simulink model "stacked_singleEMRAX_angleChange"  (R2021a)
settings: Solver=ode45  StartTime=0.0  StopTime=20  RelTol=1e-4  EnableMultiTasking=on
InitFcn:
  | %Atmospheric Properties
  | rho_air = 1.2754;  % air density in kg/m^3
  | mu = 1.803e-5; % dynamic viscosity [N-s/m^2]
  | 
  | Vbus = 175;  % Actual bus voltage (volts) that will be applied
  | % Emrax 208
  | R = .0122;  %  resistance, ohms, line-line at room temp
  | L = 125*10^-6;  %  inductance line-line at commutation frequency, henries
  | t_elec = L/R;
  | 
  | Irotor = 256/100^2;  %  kg*m^2 -- From Emrax data sheet
  | Kt_motor = .80;  %  N*m/Arms
  | Ke_motor = .0487*sqrt(2)*60/(2*pi);  %  Vpk/rad/sec
  | Ke = .0487*sqrt(2)*60/(2*pi);   %radians/sec
  | 
  | CurrentSenseMax = 250;  %  Max current sense from controller code
  | BASE_CURRENT = 125;   %  Max current in amps corresponding to normalized control loop current = 1
  | LOOP_FREQUENCY = 35;     % in kHz
  | T_LOOP = .001/LOOP_FREQUENCY;
  | pwm_loop_prescalar = 1;  %Presacalar how many PWM cycles for one current loop execution
  | T_PWM = T_LOOP/pwm_loop_prescalar;  %  Current loop prescaler on PWM is 1 for Uber
  | POLES = 20;
  | BASE_FREQ = 1200; %POLES/2*1300/60;  %  1300 rpm
  | BaseSpeed     = BASE_FREQ*(60.0/(POLES/2.0));
  | 
  | % current loop
  | alpha = 250*2*pi;         % current loop bandwidth
  | 
  | omega = 0;               % omega for de-coupling integrator
  | 
  | % Current loop
  | %          Motor_Params.ILOOP_BW = (2*PI*1000.0);
  | %        Motor_Params.id_KP = Motor_Params.ILOOP_BW*Motor_Params.StatorInductance;
  | %      Motor_Params.id_KI = Motor_Params.ILOOP_BW*Motor_Params.StatorResistance;
  | %      Motor_Params.iq_KP = Motor_Params.ILOOP_BW*Motor_Params.StatorInductance;
  | %     Motor_Params.iq_KI = Motor_Params.ILOOP_BW*Motor_Params.StatorResistance;
  | I_Kp = alpha*L*1;
  | I_Ki = alpha*R/I_Kp*T_LOOP;
  | %I_Ki = alpha*R*0;
  | 
  | % Speed loop
  | SpeedLoopPrescale = 5;
  | Tspeedloop = T_LOOP*SpeedLoopPrescale;
  | PID_spd_Kp = 3;   % From Uber code (ORIGINIAL: 3)
  | PID_spd_Ki = .15*Tspeedloop*1.5;   % From Uber code (ORIGINAL: 0.15*Tspeedloop*2)
  | 
  | Ramp_secs = 100;    %  Ramp slew rate limiter, this number is the number of seconds to ramp from 0 to basespeed
  | 
  | % Position loop
  | speedErrorPEngage = .003; % Speed error max for position loop to enable
  | % Code has .001 for PEngage, trying something diff here
  | PID_pos_Kp = .25;
  | PID_pos_Ki = .00003;
  | PID_pos_Kd = 20000;
  | 
  | PID_pos_error_sat = .3;  % Maximum error saturated into position PID (in simulink, not C right now)
  | PID_pos_sat = .25;  %  From code, based on DC bus limit
  | PID_pos_C1 = 1; %  Position loop D bandlimit filter
  | PID_pos_C2 = 0;  %  Position loop D bandlimit filter
  | 
  | 
  | % transfer function of speed estimator is K1*K3*z/(z-K2)
  | %  Pole is at z = K2
  | % z = exp(-sT)
  | f_estpole = 35000;
  | K1 = 1/(BASE_FREQ*T_LOOP);   %  Divide by base freq to convert from elec delta-normalized-angle/cycle to [0,1] normalized speed
  |      %  K1 converts delta angle estimate over a loop period to a [0,1] speed estimate
  | K2 = exp(-f_estpole*2*pi*T_LOOP);
  | K3 = 1 - K2;  % Set to make filter have unity gain at 0 frequency (z = 1)
  | 
  | %Blade properties
  | d_prop = 2.216;   %  diameter propeller [m]
  | Cp = 11000/rho_air/d_prop^5/(1300/60*2*pi)^3;   % 11000 W at 1300 rpm static thrust
  | cla = 5.73; %local lift slope [/rad] ASSUMED CONSTANT
  | cd = 0.01; %local drag coeff. ASSUMED CONSTANT
  | c = 0.08; %chord [m]
  | nb = 2; %number of blades
  | sigma = nb*c/pi/(d_prop/2);
  | Ihub = 0.0143;
  | Iblade = 0.1275;
  | Idrive = 0.0052;
  | Iloadcell = 0.011;
  | Irotorshaft = 0.0076;
  | GR = 1.6; %gear ratio
  | Ielements = Ihub*2 + Iblade*nb + Iloadcell*2;
  | I_eff = Ielements*(1/GR)^2;
  | Iload = I_eff + Idrive;   % .33 Jayant email 3/6/2019 ;  .2 jayant email 7/11/2018
  | 
  | 
  | 
  | InitialRPM = 1920;
  | omegamech = InitialRPM/60*2*pi;  %  Used to preload Q current voltage integrator
  | 
  | % Serial Message frequency (messages per second)
  | MsgFreq = 1000;
undefined symbols (not defined in the file): DiscIntNeverNeededParam, magnitude
settings Model: ModifiedHistory=4/7/2020 Adding in voltage saturation to mag 1 before SVGEN  Creator=mricci  LastModifiedBy=asper101
settings SolverCC: AlgebraicLoopSolver=TrustRegion
settings DataIOCC: LimitDataPoints=on  SaveFormat=Array  SignalLoggingSaveFormat=ModelDataLogs  ReturnWorkspaceOutputs=off
settings OptimizationCC: ExpressionDepthLimit=2147483647  InitFltsAndDblsToZero=on  LifeSpan=inf
settings DebuggingCC: UnderspecifiedInitializationDetection=Classic  MergeDetectMultiDrivingBlocksExec=none  SolverPrmCheckMsg=warning  FcnCallInpInsideContextMsg=warning  StateNameClashWarn=warning  SFUnexpectedBacktrackingDiag=warning  SFNoUnconditionalDefaultTransitionDiag=warning  SFExecutionAtInitializationDiag=none  SFMachineParentedDataDiag=warning  ArithmeticOperatorsInVariantConditions=warning
settings HardwareCC: ProdBitPerPointer=32  ProdBitPerSizeT=32  ProdBitPerPtrDiffT=32  ProdLargestAtomicFloat=None  ProdIntDivRoundTo=Undefined  ProdEndianess=Unspecified  ProdWordSize=32  ProdHWDeviceType=32-bit Generic
settings ModelReferenceCC: PropagateSignalLabelsOutOfModel=off
settings CodeAppCC: StateflowObjectComments=on
settings GRTTargetCC: TargetLangStandard=C89/C90 (ANSI)  CombineOutputUpdateFcns=off  GRTInterface=on
settings ConfigComp: CovMetricSettings=dw  CovSaveCumulativeToWorkspaceVar=on  CovSaveSingleToWorkspaceVar=on

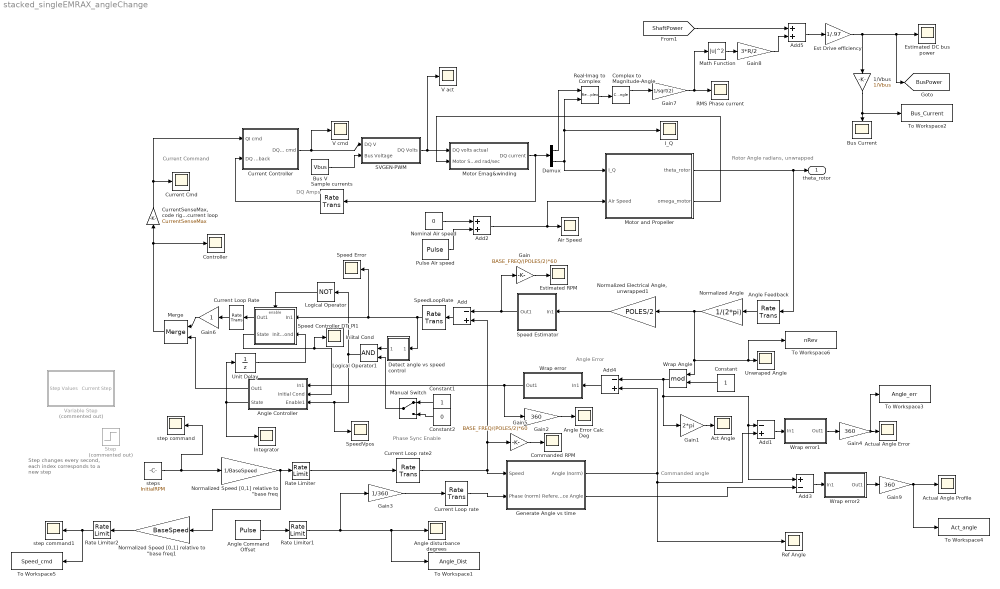
== system stacked_singleEMRAX_angleChange ==
  note: Phase Sync Enable
  note: Current Command
  note: Rotor Angle radians, unwrapped
  note: Commanded angle
  note: Angle Error
  note: DQ Amps
  note: Step changes every second, each index corresponds to a new step
  1/Vbus : Gain  Gain=1/Vbus
  Act Angle : Scope
  Actual Angle Error : Scope
  Actual Angle Profile : Scope
  Add : Sum  Inputs=-+
  Add1 : Sum  Inputs=-+
  Add2 : Sum
  Add3 : Sum  Inputs=+-
  Add4 : Sum  Inputs=-+
  Add5 : Sum
  Air Speed : Scope
  Angle Command Offset : DiscretePulseGenerator  PulseType=Time based  Amplitude=5  Period=6  PulseWidth=50  PhaseDelay=10
  Angle Controller : Subsystem  TreatAsAtomicUnit=on
  Angle Error Calc Deg : Scope
  Angle Feedback : RateTransition  OutPortSampleTime=T_LOOP
  Angle disturbance degrees : Scope
  Bus Current : Scope
  Bus V : Constant  Value=Vbus
  Commanded RPM : Scope
  Complex to Magnitude-Angle : ComplexToMagnitudeAngle
  Constant : Constant
  Constant1 : Constant
  Constant2 : Constant  Value=0
  Controller : Scope
  Current Loop Rate : RateTransition  OutPortSampleTime=T_LOOP
  Current Cmd : Scope
  Current Controller : Subsystem
  Current Loop rate : RateTransition  OutPortSampleTime=T_LOOP
  Current Loop rate2 : RateTransition  OutPortSampleTime=T_LOOP
  "CurrentSenseMax, code right now has Controller outputting PU amps then scaled to amps going into current loop" : Gain  Gain=CurrentSenseMax
  Demux : Demux  Outputs=2
  Detect angle vs speed control : Subsystem
  Est Drive efficiency : Gain  Gain=1/.97
  Estimated DC bus power : Scope
  Estimated RPM : Scope
  Gain : Gain  Gain=BASE_FREQ/(POLES/2)*60
  Gain1 : Gain  Gain=2*pi
  Gain2 : Gain  Gain=360
  Gain3 : Gain  Gain=1/360
  Gain4 : Gain  Gain=360
  Gain5 : Gain  Gain=BASE_FREQ/(POLES/2)*60
  Gain6 : Gain
  Gain7 : Gain  Gain=1/sqrt(2)
  Gain8 : Gain  Gain=3*R/2
  Gain9 : Gain  Gain=360
  Generate Angle vs time : Subsystem
  I_Q : Scope
  Iniital Cond : Scope
  Integrator : Scope
  Logical Operator : Logic  Operator=NOT  AllPortsSameDT=off  OutDataTypeStr=boolean
  Logical Operator1 : Logic  AllPortsSameDT=off  OutDataTypeStr=boolean
  Manual Switch : ManualSwitch
  Math Function : Math  Operator=magnitude^2  SaturateOnIntegerOverflow=on
  Merge : Merge
  Motor Emag&winding : Subsystem
  Motor and Propeller : Subsystem
  Nominal Air speed : Constant  Value=0
  Normalized Angle : Gain  Gain=1/(2*pi)
  "Normalized Electrical Angle, unwrapped1" : Gain  Gain=POLES/2
  "Normalized Speed [0,1] relative to \"base freq" : Gain  Gain=1/BaseSpeed
  "Normalized Speed [0,1] relative to \"base freq1" : Gain  Gain=BaseSpeed
  Pulse Air speed : DiscretePulseGenerator  PulseType=Time based  Amplitude=0  Period=6  PulseWidth=50
  RMS Phase current : Scope
  Rate Limiter : RateLimiter  RisingSlewLimit=5/Ramp_secs  FallingSlewLimit=-5/Ramp_secs  SampleTimeMode=inherited  InitialCondition=InitialRPM/BaseSpeed
  Rate Limiter1 : RateLimiter  RisingSlewLimit=5/.1  FallingSlewLimit=-5/.1  SampleTimeMode=inherited
  Rate Limiter2 : RateLimiter  RisingSlewLimit=5/Ramp_secs  FallingSlewLimit=-5/Ramp_secs  SampleTimeMode=inherited  InitialCondition=InitialRPM/BaseSpeed
  Real-Imag to Complex : RealImagToComplex
  Ref Angle : Scope
  SVGEN-PWM : Subsystem
  Sample currents : RateTransition  OutPortSampleTime=T_LOOP
  Speed Controller DT_PI1 : Subsystem
  Speed Error : Scope
  Speed Estimator : Subsystem
  SpeedLoopRate : RateTransition  OutPortSampleTime=T_LOOP*SpeedLoopPrescale
  SpeedVpos : Scope
  Step : Step  Commented=on  Time=.25  Before=InitialRPM  After=1280
  To Workspace1 : ToWorkspace  VariableName=Angle_Dist  SaveFormat=Timeseries  SampleTime=-1
  To Workspace2 : ToWorkspace  VariableName=Bus_Current  SaveFormat=Timeseries  SampleTime=-1
  To Workspace3 : ToWorkspace  VariableName=Angle_err  SaveFormat=Timeseries  SampleTime=-1
  To Workspace4 : ToWorkspace  VariableName=Act_angle  SaveFormat=Timeseries  SampleTime=-1
  To Workspace5 : ToWorkspace  VariableName=Speed_cmd  SaveFormat=Timeseries  SampleTime=-1
  To Workspace6 : ToWorkspace  VariableName=nRev  SaveFormat=Timeseries  SampleTime=-1
  Unit Delay : UnitDelay
  Unwraped Angle : Scope
  V act : Scope
  V cmd : Scope
  Variable Step : Subsystem  Commented=on
  Wrap Angle : Math  Operator=mod  SignedPower=on  SaturateOnIntegerOverflow=on
  Wrap error : Subsystem
  Wrap error1 : Subsystem
  Wrap error2 : Subsystem
  step command : Scope
  step command1 : Scope
  steps : Constant  Value=InitialRPM
  theta_rotor : Outport
  tag scope: BusPower=global
  wires:
  Motor and Propeller/1(theta_rotor) -> theta_rotor/1, Angle Feedback/1
  Add/1 -> SpeedLoopRate/1
  Speed Estimator/1(Out1) -> Add/1, Gain/1
  Add2/1 -> Air Speed/1, Motor and Propeller/2(Air Speed)
  Nominal Air speed/1 -> Add2/1
  Pulse Air speed/1 -> Add2/2
  Gain/1 -> Estimated RPM/1
  Wrap Angle/1 -> Add4/1, Gain1/1, Add3/1, Add1/1
  Constant/1 -> Wrap Angle/2
  Generate Angle vs time/1(Angle (norm)) -> Add1/2, Ref Angle/1, Add4/2
  Wrap error/1(Out1) -> Gain2/1, Angle Controller/1(In1)
  Add4/1 -> Wrap error/1(In1)
  Angle Command Offset/1 -> Rate Limiter1/1
  Speed Controller DT_PI1/1(Out1) -> Current Loop Rate/1
  Merge/1 -> "CurrentSenseMax, code right now has Controller outputting PU amps then scaled to amps going into current loop"/1, Controller/1
  SpeedLoopRate/1 -> Speed Controller DT_PI1/1(In1), Speed Error/1, Detect angle vs speed control/1(In1)
  "CurrentSenseMax, code right now has Controller outputting PU amps then scaled to amps going into current loop"/1 -> Current Controller/1(QI cmd), Current Cmd/1
  Logical Operator1/1 -> Logical Operator/1, Angle Controller/3(Enable1), SpeedVpos/1
  Motor and Propeller/2(omega_motor) -> Motor Emag&winding/2(Motor Speed rad/sec)
  Current Loop rate/1 -> Generate Angle vs time/2(Phase (norm))
  Sample currents/1 -> Current Controller/2(DQ I feedback)
  Motor Emag&winding/1(DQ current) -> Demux/1, Sample currents/1
  Demux/2 -> Real-Imag to Complex/2, I_Q/1, Motor and Propeller/1(I_Q)
  Angle Feedback/1 -> Normalized Angle/1
  Normalized Angle/1 -> "Normalized Electrical Angle, unwrapped1"/1, To Workspace6/1, Unwraped Angle/1, Wrap Angle/1
  Angle Controller/1(Out1) -> Merge/2
  "Normalized Electrical Angle, unwrapped1"/1 -> Speed Estimator/1(In1)
  Gain1/1 -> Act Angle/1
  Gain3/1 -> Current Loop rate/1
  Gain2/1 -> Angle Error Calc Deg/1
  Add1/1 -> Wrap error1/1(In1)
  Wrap error1/1(Out1) -> Gain4/1
  Gain4/1 -> To Workspace3/1, Actual Angle Error/1
  Current Loop rate2/1 -> Generate Angle vs time/1(Speed), Add/2, Gain5/1
  Angle Controller/2(State) -> Unit Delay/1, Integrator/1
  Speed Controller DT_PI1/2(State) -> Angle Controller/2(Initial Cond), Iniital Cond/1
  Gain5/1 -> Commanded RPM/1
  Current Loop Rate/1 -> Gain6/1
  Gain6/1 -> Merge/1
  Logical Operator/1 -> Speed Controller DT_PI1/Enable
  Current Controller/1(DQ V cmd) -> SVGEN-PWM/1(DQ V), V cmd/1
  SVGEN-PWM/1(DQ Volts) -> V act/1, Motor Emag&winding/1(DQ volts actual)
  Bus V/1 -> SVGEN-PWM/2(Bus Voltage)
  Unit Delay/1 -> Speed Controller DT_PI1/2(Initial Cond)
  Rate Limiter/1 -> Current Loop rate2/1
  Detect angle vs speed control/1(Out1) -> Logical Operator1/1
  Manual Switch/1 -> Logical Operator1/2
  Constant1/1 -> Manual Switch/1
  Constant2/1 -> Manual Switch/2
  "Normalized Speed [0,1] relative to \"base freq"/1 -> "Normalized Speed [0,1] relative to \"base freq1"/1, Rate Limiter/1
  Demux/1 -> Real-Imag to Complex/1
  Real-Imag to Complex/1 -> Complex to Magnitude-Angle/1
  Complex to Magnitude-Angle/1 -> Gain7/1
  Gain7/1 -> Math Function/1, RMS Phase current/1
  [ShaftPower] -> Add5/1
  Math Function/1 -> Gain8/1
  Gain8/1 -> Add5/2
  Add5/1 -> Est Drive efficiency/1
  Est Drive efficiency/1 -> 1/Vbus/1, [BusPower], Estimated DC bus power/1
  1/Vbus/1 -> To Workspace2/1, Bus Current/1
  Gain9/1 -> To Workspace4/1, Actual Angle Profile/1
  Wrap error2/1(Out1) -> Gain9/1
  Add3/1 -> Wrap error2/1(In1)
  Generate Angle vs time/2(Reference Angle) -> Add3/2
  Rate Limiter1/1 -> Gain3/1, Angle disturbance degrees/1, To Workspace1/1
  "Normalized Speed [0,1] relative to \"base freq1"/1 -> Rate Limiter2/1
  Rate Limiter2/1 -> To Workspace5/1, step command1/1
  steps/1 -> step command/1, "Normalized Speed [0,1] relative to \"base freq"/1

== system stacked_singleEMRAX_angleChange/Angle Controller ==
  In1 : Inport
  Initial Cond : Inport  Port=2
  Enable1 : Inport  Port=3
  Angle Controller DT_PID saturate P : Subsystem
  Max error : Saturate  UpperLimit=PID_pos_error_sat  LowerLimit=-PID_pos_error_sat
  Out1 : Outport  InitialOutput=[0]
  State : Outport  Port=2  InitialOutput=[0]
  wires:
  In1/1 -> Max error/1
  Max error/1 -> Angle Controller DT_PID saturate P/1(In1)
  Initial Cond/1 -> Angle Controller DT_PID saturate P/2(Iniitial Cond)
  Enable1/1 -> Angle Controller DT_PID saturate P/Enable
  Angle Controller DT_PID saturate P/1(Out1) -> Out1/1
  Angle Controller DT_PID saturate P/2(Integrator) -> State/1

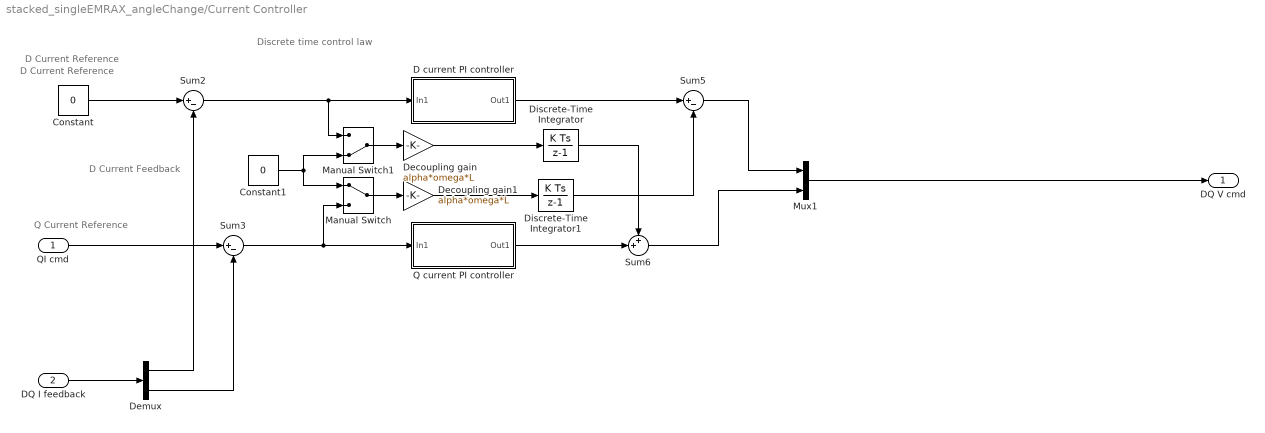
== system stacked_singleEMRAX_angleChange/Current Controller ==
  note: D Current Reference
  note: D Current Feedback
  note: D Current Reference
  note: Q Current Reference
  note: Discrete
      | time control
      | law
  QI cmd : Inport
  DQ I feedback : Inport  Port=2
  Constant : Constant  Value=0
  Constant1 : Constant  Value=0
  D current PI controller : Subsystem
  Decoupling gain : Gain  Gain=alpha*omega*L
  Decoupling gain1 : Gain  Gain=alpha*omega*L
  Demux : Demux  Outputs=2
  Discrete-Time Integrator : DiscreteIntegrator  SampleTime=T_LOOP  ICPrevOutput=DiscIntNeverNeededParam  ICPrevScaledInput=DiscIntNeverNeededParam
  Discrete-Time Integrator1 : DiscreteIntegrator  SampleTime=T_LOOP  ICPrevOutput=DiscIntNeverNeededParam  ICPrevScaledInput=DiscIntNeverNeededParam
  Manual Switch : ManualSwitch
  Manual Switch1 : ManualSwitch  CurrentSetting=0
  Mux1 : Mux  Inputs=2
  Q current PI controller : Subsystem
  Sum2 : Sum  Inputs=|+-
  Sum3 : Sum  Inputs=|+-
  Sum5 : Sum  Inputs=|+-
  Sum6 : Sum  Inputs=++|
  DQ V cmd : Outport
  wires:
  Mux1/1 -> DQ V cmd/1
  Sum2/1 -> D current PI controller/1(In1), Manual Switch1/1
  Sum3/1 -> Q current PI controller/1(In1), Manual Switch/2
  Constant/1 -> Sum2/1
  D current PI controller/1(Out1) -> Sum5/1
  Q current PI controller/1(Out1) -> Sum6/2
  Discrete-Time Integrator/1 -> Sum6/1
  Discrete-Time Integrator1/1 -> Sum5/2
  QI cmd/1 -> Sum3/1
  Decoupling gain1/1 -> Discrete-Time Integrator1/1
  Decoupling gain/1 -> Discrete-Time Integrator/1
  Manual Switch/1 -> Decoupling gain1/1
  Manual Switch1/1 -> Decoupling gain/1
  Constant1/1 -> Manual Switch1/2, Manual Switch/1
  Sum5/1 -> Mux1/1
  Sum6/1 -> Mux1/2
  DQ I feedback/1 -> Demux/1
  Demux/1 -> Sum2/2
  Demux/2 -> Sum3/2

== system stacked_singleEMRAX_angleChange/Detect angle vs speed control ==
  In1 : Inport
  Abs : Abs
  Relay : Relay  OnSwitchValue=2*speedErrorPEngage  OffSwitchValue=speedErrorPEngage  OnOutputValue=0  OffOutputValue=1
  Out1 : Outport
  wires:
  Abs/1 -> Relay/1
  In1/1 -> Abs/1
  Relay/1 -> Out1/1

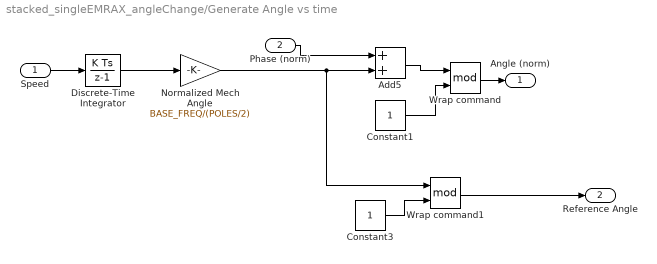
== system stacked_singleEMRAX_angleChange/Generate Angle vs time ==
  Speed : Inport
  Phase (norm) : Inport  Port=2
  Add5 : Sum
  Constant1 : Constant
  Constant3 : Constant
  Discrete-Time Integrator : DiscreteIntegrator  SampleTime=-1  ICPrevOutput=DiscIntNeverNeededParam  ICPrevScaledInput=DiscIntNeverNeededParam
  Normalized Mech Angle : Gain  Gain=BASE_FREQ/(POLES/2)
  Wrap command : Math  Operator=mod  SignedPower=on  SaturateOnIntegerOverflow=on
  Wrap command1 : Math  Operator=mod  SignedPower=on  SaturateOnIntegerOverflow=on
  Angle (norm) : Outport
  Reference Angle : Outport  Port=2
  wires:
  Constant1/1 -> Wrap command/2
  Discrete-Time Integrator/1 -> Normalized Mech Angle/1
  Add5/1 -> Wrap command/1
  Speed/1 -> Discrete-Time Integrator/1
  Phase (norm)/1 -> Add5/1
  Wrap command/1 -> Angle (norm)/1
  Constant3/1 -> Wrap command1/2
  Normalized Mech Angle/1 -> Wrap command1/1, Add5/2
  Wrap command1/1 -> Reference Angle/1

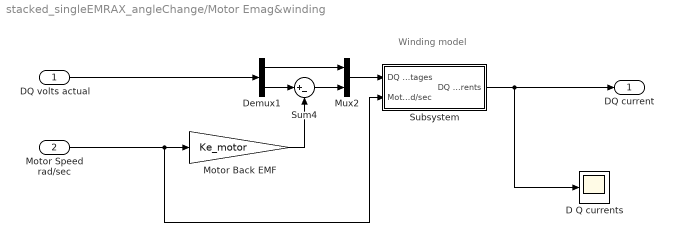
== system stacked_singleEMRAX_angleChange/Motor Emag&winding ==
  note: Winding model
  DQ volts actual : Inport
  Motor Speed rad/sec : Inport  Port=2
  D Q currents : Scope
  Demux1 : Demux  Outputs=2
  Motor Back EMF : Gain  Gain=Ke_motor
  Mux2 : Mux  Inputs=2
  Subsystem : Subsystem
  Sum4 : Sum  Inputs=|+-
  DQ current : Outport
  wires:
  Motor Speed rad/sec/1 -> Motor Back EMF/1, Subsystem/2(Motor speed rad/sec)
  Mux2/1 -> Subsystem/1(DQ voltages)
  Demux1/1 -> Mux2/1
  Demux1/2 -> Sum4/1
  Sum4/1 -> Mux2/2
  Motor Back EMF/1 -> Sum4/2
  DQ volts actual/1 -> Demux1/1
  Subsystem/1(DQ currents) -> DQ current/1, D Q currents/1

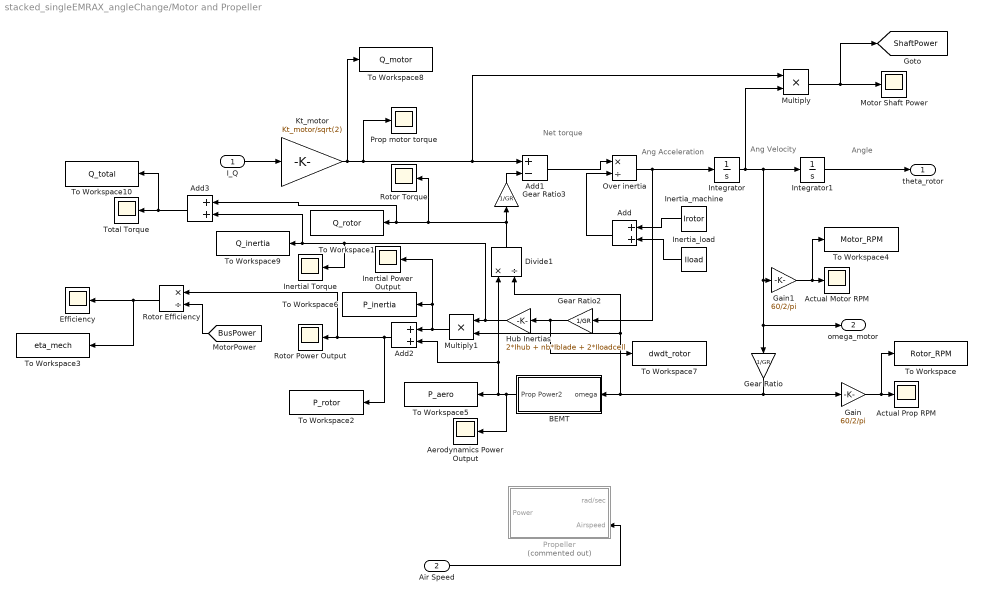
== system stacked_singleEMRAX_angleChange/Motor and Propeller ==
  note: Ang Acceleration
  note: Angle
  note: Ang Velocity
  note: Net torque
  I_Q : Inport
  Air Speed : Inport  Port=2
  Actual Motor RPM : Scope
  Actual Prop RPM : Scope
  Add : Sum
  Add1 : Sum  Inputs=+-
  Add2 : Sum
  Add3 : Sum
  Aerodynamics Power Output : Scope
  BEMT : Subsystem
  Divide1 : Product  Inputs=*/
  Efficiency : Scope
  Gain : Gain  Gain=60/2/pi
  Gain1 : Gain  Gain=60/2/pi
  Gear Ratio : Gain  Gain=1/GR
  Gear Ratio2 : Gain  Gain=1/GR
  Gear Ratio3 : Gain  Gain=1/GR
  Hub Inertias : Gain  Gain=2*Ihub + nb*Iblade + 2*Iloadcell
  Inertia_load : Constant  Value=Iload
  Inertia_machine : Constant  Value=Irotor
  Inertial Power Output : Scope
  Inertial Torque : Scope
  Integrator : Integrator  InitialCondition=InitialRPM*2*pi/60
  Integrator1 : Integrator
  Kt_motor : Gain  Gain=Kt_motor/sqrt(2)
  Motor Shaft Power : Scope
  Multiply : Product  Inputs=**
  Multiply1 : Product  Inputs=**
  Over inertia : Product  Inputs=*/
  Prop motor torque : Scope
  Propeller : Subsystem  Commented=on
  Rotor Efficiency : Product  Inputs=*/
  Rotor Power Output : Scope
  Rotor Torque : Scope
  To Workspace : ToWorkspace  VariableName=Rotor_RPM  SaveFormat=Timeseries  SampleTime=-1
  To Workspace1 : ToWorkspace  VariableName=Q_rotor  SaveFormat=Timeseries  SampleTime=-1
  To Workspace10 : ToWorkspace  VariableName=Q_total  SaveFormat=Timeseries  SampleTime=-1
  To Workspace2 : ToWorkspace  VariableName=P_rotor  SaveFormat=Timeseries  SampleTime=-1
  To Workspace3 : ToWorkspace  VariableName=eta_mech  SaveFormat=Timeseries  SampleTime=-1
  To Workspace4 : ToWorkspace  VariableName=Motor_RPM  SaveFormat=Timeseries  SampleTime=-1
  To Workspace5 : ToWorkspace  VariableName=P_aero  SaveFormat=Timeseries  SampleTime=-1
  To Workspace6 : ToWorkspace  VariableName=P_inertia  SaveFormat=Timeseries  SampleTime=-1
  To Workspace7 : ToWorkspace  VariableName=dwdt_rotor  SaveFormat=Timeseries  SampleTime=-1
  To Workspace8 : ToWorkspace  VariableName=Q_motor  SaveFormat=Timeseries  SampleTime=-1
  To Workspace9 : ToWorkspace  VariableName=Q_inertia  SaveFormat=Timeseries  SampleTime=-1
  Total Torque : Scope
  theta_rotor : Outport
  omega_motor : Outport  Port=2
  tag scope: ShaftPower=global
  wires:
  Integrator/1 -> Integrator1/1, Gain1/1, omega_motor/1, Gear Ratio/1, Multiply/2
  I_Q/1 -> Kt_motor/1
  Air Speed/1 -> Propeller/2(Airspeed)
  Over inertia/1 -> Gear Ratio2/1, Integrator/1
  Integrator1/1 -> theta_rotor/1
  Add1/1 -> Over inertia/1
  Kt_motor/1 -> Multiply/1, Add1/1, Prop motor torque/1, To Workspace8/1
  Gain/1 -> To Workspace/1, Actual Prop RPM/1
  Inertia_machine/1 -> Add/1
  Inertia_load/1 -> Add/2
  Add/1 -> Over inertia/2
  Multiply/1 -> [ShaftPower], Motor Shaft Power/1
  Gear Ratio/1 -> Divide1/2, Multiply1/2, BEMT/1(omega), Gain/1
  BEMT/1(Prop Power2) -> Aerodynamics Power Output/1, Add2/2, Divide1/1, To Workspace5/1
  Rotor Efficiency/1 -> To Workspace3/1, Efficiency/1
  Gain1/1 -> To Workspace4/1, Actual Motor RPM/1
  [BusPower] -> Rotor Efficiency/2
  Add2/1 -> Rotor Efficiency/1, Rotor Power Output/1, To Workspace2/1
  Gear Ratio2/1 -> To Workspace7/1, Hub Inertias/1
  Gear Ratio3/1 -> Add1/2
  Divide1/1 -> Rotor Torque/1, Add3/1, To Workspace1/1, Gear Ratio3/1
  Hub Inertias/1 -> Inertial Torque/1, Add3/2, To Workspace9/1, Multiply1/1
  Multiply1/1 -> Inertial Power Output/1, To Workspace6/1, Add2/1
  Add3/1 -> To Workspace10/1, Total Torque/1

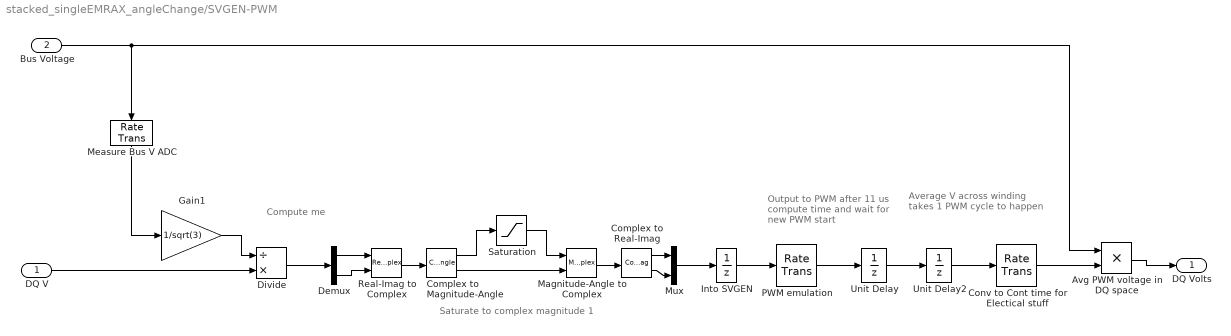
== system stacked_singleEMRAX_angleChange/SVGEN-PWM ==
  note: Saturate to complex magnitude 1
  note: Output to PWM
      | after 11 us compute time
      | and wait for new PWM start
  note: Average V
      | across winding
      | takes 1 PWM
      | cycle to happen
  note: Compute
      | me
  DQ V : Inport
  Bus Voltage : Inport  Port=2
  Avg PWM voltage in DQ space : Product  RndMeth=Zero
  Complex to Magnitude-Angle : ComplexToMagnitudeAngle
  Complex to Real-Imag : ComplexToRealImag
  Conv to Cont time for Electical stuff : RateTransition
  Demux : Demux  Outputs=2
  Divide : Product  Inputs=/*
  Gain1 : Gain  Gain=1/sqrt(3)
  Into SVGEN : UnitDelay  InitialCondition=[ 0 ; omegamech*Ke/Vbus]  SampleTime=-1
  Magnitude-Angle to Complex : MagnitudeAngleToComplex
  Measure Bus V ADC : RateTransition  OutPortSampleTime=T_LOOP
  Mux : Mux  Inputs=2
  PWM emulation : RateTransition  OutPortSampleTime=T_PWM
  Real-Imag to Complex : RealImagToComplex
  Saturation : Saturate  UpperLimit=1  LowerLimit=-1
  Unit Delay : UnitDelay  InitialCondition=[ 0 ; omegamech*Ke/Vbus]  SampleTime=-1
  Unit Delay2 : UnitDelay  InitialCondition=[ 0 ; omegamech*Ke/Vbus]  SampleTime=-1
  DQ Volts : Outport
  wires:
  Into SVGEN/1 -> PWM emulation/1
  Unit Delay/1 -> Unit Delay2/1
  PWM emulation/1 -> Unit Delay/1
  Unit Delay2/1 -> Conv to Cont time for Electical stuff/1
  Bus Voltage/1 -> Measure Bus V ADC/1, Avg PWM voltage in DQ space/1
  Measure Bus V ADC/1 -> Gain1/1
  Gain1/1 -> Divide/1
  DQ V/1 -> Divide/2
  Conv to Cont time for Electical stuff/1 -> Avg PWM voltage in DQ space/2
  Avg PWM voltage in DQ space/1 -> DQ Volts/1
  Mux/1 -> Into SVGEN/1
  Divide/1 -> Demux/1
  Demux/1 -> Real-Imag to Complex/1
  Demux/2 -> Real-Imag to Complex/2
  Real-Imag to Complex/1 -> Complex to Magnitude-Angle/1
  Complex to Magnitude-Angle/1 -> Saturation/1
  Saturation/1 -> Magnitude-Angle to Complex/1
  Complex to Magnitude-Angle/2 -> Magnitude-Angle to Complex/2
  Magnitude-Angle to Complex/1 -> Complex to Real-Imag/1
  Complex to Real-Imag/1 -> Mux/1
  Complex to Real-Imag/2 -> Mux/2

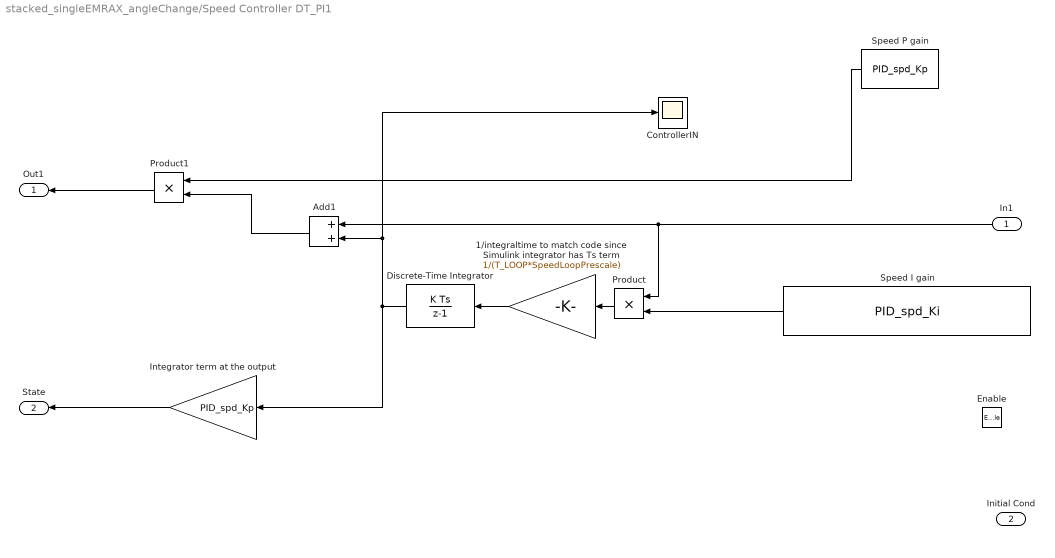
== system stacked_singleEMRAX_angleChange/Speed Controller DT_PI1 ==
  In1 : Inport
  Initial Cond : Inport  Port=2
  Enable : EnablePort  ShowOutputPort=on
  1/integraltime to match code since Simulink integrator has Ts term : Gain  Gain=1/(T_LOOP*SpeedLoopPrescale)
  Add1 : Sum
  ControllerIN : Scope
  Discrete-Time Integrator : DiscreteIntegrator  InitialCondition=.03  SampleTime=-1  ICPrevOutput=DiscIntNeverNeededParam  ICPrevScaledInput=DiscIntNeverNeededParam
  Integrator term at the output : Gain  Gain=PID_spd_Kp
  Product : Product  RndMeth=Zero
  Product1 : Product  RndMeth=Zero
  Speed I gain : Constant  Value=PID_spd_Ki
  Speed P gain : Constant  Value=PID_spd_Kp
  Out1 : Outport
  State : Outport  Port=2
  wires:
  Product/1 -> 1/integraltime to match code since Simulink integrator has Ts term/1
  In1/1 -> Product/1, Add1/1
  1/integraltime to match code since Simulink integrator has Ts term/1 -> Discrete-Time Integrator/1
  Speed I gain/1 -> Product/2
  Speed P gain/1 -> Product1/1
  Discrete-Time Integrator/1 -> Integrator term at the output/1, ControllerIN/1, Add1/2
  Add1/1 -> Product1/2
  Product1/1 -> Out1/1
  Integrator term at the output/1 -> State/1

== system stacked_singleEMRAX_angleChange/Speed Estimator ==
  In1 : Inport
  Add1 : Sum  Inputs=+-
  DeltaAngle : Scope
  Sampling : UnitDelay  SampleTime=-1
  Speed Estimator : Subsystem
  Unit Delay1 : UnitDelay  SampleTime=-1
  Out1 : Outport
  wires:
  Sampling/1 -> Add1/1, Unit Delay1/1
  Unit Delay1/1 -> Add1/2
  Add1/1 -> Speed Estimator/1(delta angle), DeltaAngle/1
  In1/1 -> Sampling/1
  Speed Estimator/1(Est Speed [0,1]) -> Out1/1

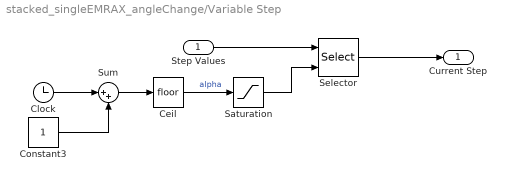
== system stacked_singleEMRAX_angleChange/Variable Step ==
  Step Values : Inport
  Ceil : Rounding
  Clock : Clock
  Constant3 : Constant
  Saturation : Saturate  UpperLimit=4  LowerLimit=-inf
  Selector : Selector  InputPortWidth=4  IndexOptions=Index vector (port)  Indices=[1 3]  OutputSizes=1
  Sum : Sum  Inputs=|++
  Current Step : Outport
  wires:
  Ceil/1 -> Saturation/1  "alpha"
  Step Values/1 -> Selector/1
  Selector/1 -> Current Step/1
  Constant3/1 -> Sum/2
  Saturation/1 -> Selector/2
  Clock/1 -> Sum/1
  Sum/1 -> Ceil/1

== system stacked_singleEMRAX_angleChange/Wrap error ==
  In1 : Inport
  Add 2pi : Subsystem  TreatAsAtomicUnit=on
  If Action Subsystem : Subsystem  TreatAsAtomicUnit=on
  If1 : If  IfExpression=u1 > .5  ElseIfExpressions=u1<-.5
  Merge : Merge  Inputs=3
  Subtract 2pi1 : Subsystem  TreatAsAtomicUnit=on
  Out1 : Outport
  wires:
  In1/1 -> Add 2pi/1(In1), If Action Subsystem/1(In1), Subtract 2pi1/1(In1), If1/1
  Subtract 2pi1/1(Out1) -> Merge/1
  Merge/1 -> Out1/1
  If1/1 -> Subtract 2pi1/Action
  If1/3 -> If Action Subsystem/Action
  Add 2pi/1(Out1) -> Merge/2
  If Action Subsystem/1(Out1) -> Merge/3
  If1/2 -> Add 2pi/Action

== system stacked_singleEMRAX_angleChange/Wrap error1 ==
  In1 : Inport
  Add 2pi : Subsystem  TreatAsAtomicUnit=on
  If Action Subsystem : Subsystem  TreatAsAtomicUnit=on
  If1 : If  IfExpression=u1 > .5  ElseIfExpressions=u1<-.5
  Merge : Merge  Inputs=3
  Subtract 2pi1 : Subsystem  TreatAsAtomicUnit=on
  Out1 : Outport
  wires:
  In1/1 -> Add 2pi/1(In1), If Action Subsystem/1(In1), Subtract 2pi1/1(In1), If1/1
  Subtract 2pi1/1(Out1) -> Merge/1
  Merge/1 -> Out1/1
  If1/1 -> Subtract 2pi1/Action
  If1/3 -> If Action Subsystem/Action
  Add 2pi/1(Out1) -> Merge/2
  If Action Subsystem/1(Out1) -> Merge/3
  If1/2 -> Add 2pi/Action

== system stacked_singleEMRAX_angleChange/Wrap error2 ==
  In1 : Inport
  Add 2pi : Subsystem  TreatAsAtomicUnit=on
  If Action Subsystem : Subsystem  TreatAsAtomicUnit=on
  If1 : If  IfExpression=u1 > .5  ElseIfExpressions=u1<-.5
  Merge : Merge  Inputs=3
  Subtract 2pi1 : Subsystem  TreatAsAtomicUnit=on
  Out1 : Outport
  wires:
  In1/1 -> Add 2pi/1(In1), If Action Subsystem/1(In1), Subtract 2pi1/1(In1), If1/1
  Subtract 2pi1/1(Out1) -> Merge/1
  Merge/1 -> Out1/1
  If1/1 -> Subtract 2pi1/Action
  If1/3 -> If Action Subsystem/Action
  Add 2pi/1(Out1) -> Merge/2
  If Action Subsystem/1(Out1) -> Merge/3
  If1/2 -> Add 2pi/Action

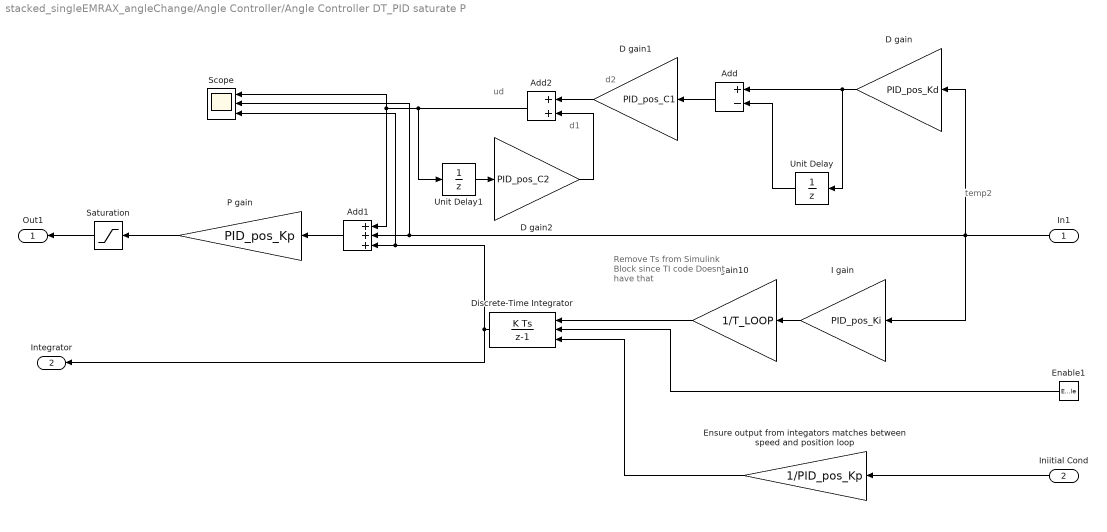
== system stacked_singleEMRAX_angleChange/Angle Controller/Angle Controller DT_PID saturate P ==
  note: Remove Ts from Simulink
      | Block since TI code
      | Doesnt have that
  note: temp2
  note: d2
  note: ud
  note: d1
  In1 : Inport
  Iniitial Cond : Inport  Port=2
  Enable1 : EnablePort  ShowOutputPort=on
  Add : Sum  Inputs=+-
  Add1 : Sum  Inputs=+++
  Add2 : Sum
  D gain : Gain  Gain=PID_pos_Kd
  D gain1 : Gain  Gain=PID_pos_C1
  D gain2 : Gain  Gain=PID_pos_C2
  Discrete-Time Integrator : DiscreteIntegrator  ExternalReset=rising  InitialConditionSource=external  SampleTime=-1  UpperSaturationLimit=BASE_CURRENT  LowerSaturationLimit=-BASE_CURRENT  ICPrevOutput=DiscIntNeverNeededParam  ICPrevScaledInput=DiscIntNeverNeededParam
  Ensure output from integators matches between speed and position loop : Gain  Gain=1/PID_pos_Kp
  I gain : Gain  Gain=PID_pos_Ki
  P gain : Gain  Gain=PID_pos_Kp
  Saturation : Saturate  UpperLimit=PID_pos_sat  LowerLimit=-PID_pos_sat
  Scope : Scope  NumInputPorts=3
  Unit Delay : UnitDelay  SampleTime=-1
  Unit Delay1 : UnitDelay  SampleTime=-1
  gain10 : Gain  Gain=1/T_LOOP
  Out1 : Outport
  Integrator : Outport  Port=2
  wires:
  Discrete-Time Integrator/1 -> Scope/3, Add1/3, Integrator/1
  I gain/1 -> gain10/1
  In1/1 -> I gain/1, Scope/2, Add1/2, D gain/1
  Add1/1 -> P gain/1
  gain10/1 -> Discrete-Time Integrator/1
  Iniitial Cond/1 -> Ensure output from integators matches between speed and position loop/1
  Unit Delay/1 -> Add/2
  P gain/1 -> Saturation/1
  Saturation/1 -> Out1/1
  D gain/1 -> Add/1, Unit Delay/1
  Add/1 -> D gain1/1
  Add2/1 -> Scope/1, Add1/1, Unit Delay1/1
  Unit Delay1/1 -> D gain2/1
  D gain2/1 -> Add2/2
  D gain1/1 -> Add2/1
  Ensure output from integators matches between speed and position loop/1 -> Discrete-Time Integrator/3
  Enable1/1 -> Discrete-Time Integrator/2

== system stacked_singleEMRAX_angleChange/Current Controller/D current PI controller ==
  In1 : Inport
  Gain : Gain  Gain=I_Kp
  Gain1 : Gain  Gain=I_Ki
  K=1/Ts DT itegrator : DiscreteIntegrator  gainval=1/T_LOOP  InitialCondition=-2  SampleTime=-1  LimitOutput=on  UpperSaturationLimit=Vbus*sqrt(3)  LowerSaturationLimit=-Vbus*sqrt(3)  ICPrevOutput=DiscIntNeverNeededParam  ICPrevScaledInput=DiscIntNeverNeededParam
  Sum : Sum  Inputs=|++
  Out1 : Outport
  wires:
  In1/1 -> Gain/1
  Gain/1 -> Sum/1, Gain1/1
  Gain1/1 -> K=1/Ts DT itegrator/1
  K=1/Ts DT itegrator/1 -> Sum/2
  Sum/1 -> Out1/1

== system stacked_singleEMRAX_angleChange/Current Controller/Q current PI controller ==
  In1 : Inport
  1/Ts gain DT integrator : DiscreteIntegrator  gainval=1/T_LOOP  InitialCondition=80  SampleTime=-1  LimitOutput=on  UpperSaturationLimit=Vbus*sqrt(3)  LowerSaturationLimit=-Vbus*sqrt(3)  ICPrevOutput=DiscIntNeverNeededParam  ICPrevScaledInput=DiscIntNeverNeededParam
  Gain : Gain  Gain=I_Kp
  Gain1 : Gain  Gain=I_Ki
  Sum : Sum  Inputs=|++
  Out1 : Outport
  wires:
  Sum/1 -> Out1/1
  1/Ts gain DT integrator/1 -> Sum/2
  Gain1/1 -> 1/Ts gain DT integrator/1
  Gain/1 -> Sum/1, Gain1/1
  In1/1 -> Gain/1

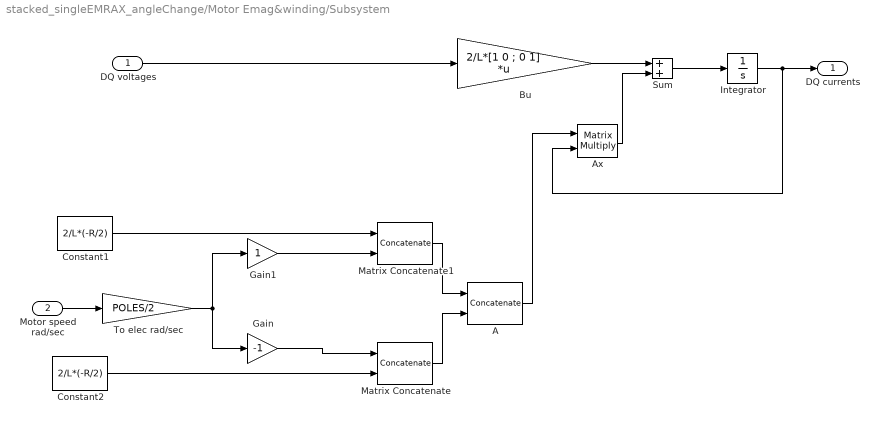
== system stacked_singleEMRAX_angleChange/Motor Emag&winding/Subsystem ==
  DQ voltages : Inport
  Motor speed rad/sec : Inport  Port=2
  A : Concatenate  Mode=Multidimensional array
  Ax : Product  Multiplication=Matrix(*)  RndMeth=Zero
  Bu : Gain  Gain=2/L*[1 0 ; 0 1]  Multiplication=Matrix(K*u)
  Constant1 : Constant  Value=2/L*(-R/2)
  Constant2 : Constant  Value=2/L*(-R/2)
  Gain : Gain  Gain=-1
  Gain1 : Gain
  Integrator : Integrator  InitialCondition=[0 25]
  Matrix Concatenate : Concatenate  Mode=Multidimensional array  ConcatenateDimension=2
  Matrix Concatenate1 : Concatenate  Mode=Multidimensional array  ConcatenateDimension=2
  Sum : Sum
  To elec rad/sec : Gain  Gain=POLES/2
  DQ currents : Outport
  wires:
  DQ voltages/1 -> Bu/1
  Integrator/1 -> DQ currents/1, Ax/2
  Sum/1 -> Integrator/1
  Bu/1 -> Sum/1
  Motor speed rad/sec/1 -> To elec rad/sec/1
  Ax/1 -> Sum/2
  A/1 -> Ax/1
  Matrix Concatenate1/1 -> A/1
  Matrix Concatenate/1 -> A/2
  Constant1/1 -> Matrix Concatenate1/1
  Constant2/1 -> Matrix Concatenate/2
  Gain1/1 -> Matrix Concatenate1/2
  To elec rad/sec/1 -> Gain1/1, Gain/1
  Gain/1 -> Matrix Concatenate/1

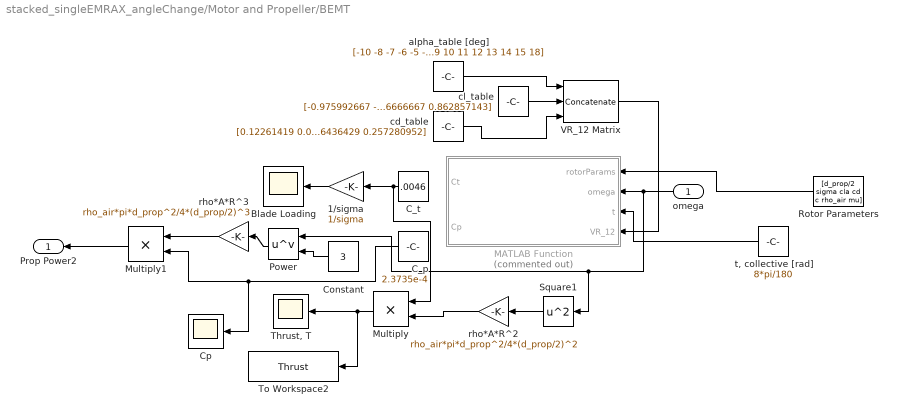
== system stacked_singleEMRAX_angleChange/Motor and Propeller/BEMT ==
  omega : Inport
  1/sigma : Gain  Gain=1/sigma
  Blade Loading : Scope
  C_p : Constant  Value=2.3735e-4
  C_t : Constant  Value=.0046
  Constant : Constant  Value=3
  Cp : Scope
  MATLAB Function : MATLAB Function  Commented=on  TreatAsAtomicUnit=on
  Multiply : Product  Inputs=**
  Multiply1 : Product  Inputs=**
  Power : Math  Operator=pow  SaturateOnIntegerOverflow=on
  Rotor Parameters : Constant  Value=[d_prop/2 sigma cla cd c rho_air mu]
  Square1 : Math  Operator=square  SaturateOnIntegerOverflow=on
  "Thrust, T" : Scope
  To Workspace2 : ToWorkspace  VariableName=Thrust  SaveFormat=Timeseries  SampleTime=-1
  VR_12 Matrix : Concatenate  NumInputs=3  Mode=Multidimensional array  ConcatenateDimension=2
  alpha_table [deg] : Constant  Value=|
      | [-10
      | -8
      | -7
      | -6
      | -5
      | -4
      | -3
      | -2
      | -1
      | 0
      | 1
      | 2
      | 3
      | 4
      | 5
      | 6
      | 7
      | 8
      | 9
      | 10
      | 11
      | 12
      | 13
      | 14
      | 15
      | 18]
  cd_table : Constant  Value=|
      | [0.12261419
      | 0.087680917
      | 0.057867958
      | 0.039199075
      | 0.029194975
      | 0.022437746
      | 0.019176417
      | 0.016951895
      | 0.016099494
      | 0.016406078
      | 0.016309381
      | 0.01677868
      | 0.017190605
      | 0.018350632
      | 0.020080972
      | 0.022798258
      | 0.028558686
      | 0.033168956
      | 0.038779694
      | 0.049736781
      | 0.069447104
      | 0.099585267
      | 0.140693562
      | 0.209493095
      | 0.226436429
      | 0.257280952]
  cl_table : Constant  Value=|
      | [-0.975992667
      | -0.829689867
      | -0.699749295
      | -0.576245171
      | -0.455593
      | -0.337596705
      | -0.208765543
      | -0.092283694
      | 0.029533567
      | 0.14688021
      | 0.269076229
      | 0.390337048
      | 0.511257305
      | 0.628967267
      | 0.744194143
      | 0.853961581
      | 0.964028571
      | 1.05643419
      | 1.13719381
      | 1.16548019
      | 1.148423714
      | 1.10768819
      | 1.011663333
      | 1.056190476
      | 1.466666667
      | 0.862857143]
  rho*A*R^2 : Gain  Gain=rho_air*pi*d_prop^2/4*(d_prop/2)^2
  rho*A*R^3 : Gain  Gain=rho_air*pi*d_prop^2/4*(d_prop/2)^3
  "t, collective [rad]" : Constant  Value=8*pi/180
  Prop Power2 : Outport
  wires:
  rho*A*R^3/1 -> Multiply1/1
  omega/1 -> Square1/1, Power/1, MATLAB Function/2(omega)
  Power/1 -> rho*A*R^3/1
  rho*A*R^2/1 -> Multiply/2
  Square1/1 -> rho*A*R^2/1
  "t, collective [rad]"/1 -> MATLAB Function/3(t)
  Multiply1/1 -> Prop Power2/1
  1/sigma/1 -> Blade Loading/1
  Rotor Parameters/1 -> MATLAB Function/1(rotorParams)
  Multiply/1 -> To Workspace2/1, "Thrust, T"/1
  Constant/1 -> Power/2
  VR_12 Matrix/1 -> MATLAB Function/4(VR_12)
  cl_table/1 -> VR_12 Matrix/2
  cd_table/1 -> VR_12 Matrix/3
  alpha_table [deg]/1 -> VR_12 Matrix/1
  C_t/1 -> Multiply/1, 1/sigma/1
  C_p/1 -> Multiply1/2, Cp/1

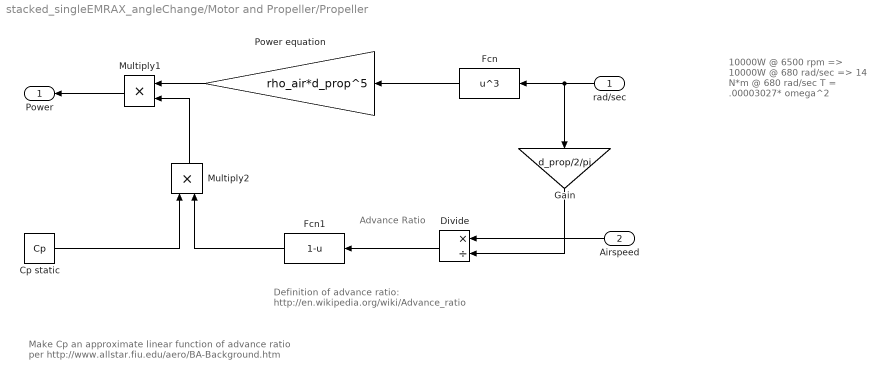
== system stacked_singleEMRAX_angleChange/Motor and Propeller/Propeller ==
  note: 10000W @ 6500 rpm =>
      | 10000W @ 680 rad/sec =>
      | 14 N*m @ 680 rad/sec
      | T =   .00003027* omega^2
  note: Make Cp an approximate
      | linear function of advance ratio
      | per http://www.allstar.fiu.edu/aero/BA-Background.htm
  note: Advance Ratio
  note: Definition of advance ratio:
      | http://en.wikipedia.org/wiki/Advance_ratio
  rad/sec : Inport
  Airspeed : Inport  Port=2
  Cp static : Constant  Value=Cp
  Divide : Product  Inputs=*/
  Fcn : Fcn  Expr=u^3
  Fcn1 : Fcn  Expr=1-u
  Gain : Gain  Gain=d_prop/2/pi
  Multiply1 : Product  Inputs=**
  Multiply2 : Product  Inputs=**
  Power equation : Gain  Gain=rho_air*d_prop^5
  Power : Outport
  wires:
  Fcn/1 -> Power equation/1
  rad/sec/1 -> Fcn/1, Gain/1
  Airspeed/1 -> Divide/1
  Gain/1 -> Divide/2
  Power equation/1 -> Multiply1/1
  Multiply1/1 -> Power/1
  Multiply2/1 -> Multiply1/2
  Cp static/1 -> Multiply2/1
  Divide/1 -> Fcn1/1
  Fcn1/1 -> Multiply2/2

== system stacked_singleEMRAX_angleChange/Speed Estimator/Speed Estimator ==
  delta angle : Inport
  Add1 : Sum  SampleTime=T_LOOP
  Filter gain for unity at 0 freq : Gain  Gain=K3
  Set filer pole : Gain  Gain=K2
  Unit Delay1 : UnitDelay  InitialCondition=.021  SampleTime=T_LOOP
  "[0,1] normalization unfiltered speed est from delta angle" : Gain  Gain=K1
  Est Speed [0,1] : Outport
  wires:
  delta angle/1 -> "[0,1] normalization unfiltered speed est from delta angle"/1
  Filter gain for unity at 0 freq/1 -> Add1/1
  Add1/1 -> Est Speed [0,1]/1, Unit Delay1/1
  Set filer pole/1 -> Add1/2
  Unit Delay1/1 -> Set filer pole/1
  "[0,1] normalization unfiltered speed est from delta angle"/1 -> Filter gain for unity at 0 freq/1

== system stacked_singleEMRAX_angleChange/Wrap error/Add 2pi ==
  In1 : Inport
  Action Port : ActionPort  ActionPortLabel=elseif(u1<-.5)
  Add5 : Sum
  Constant2 : Constant
  Out1 : Outport
  wires:
  In1/1 -> Add5/1
  Add5/1 -> Out1/1
  Constant2/1 -> Add5/2

== system stacked_singleEMRAX_angleChange/Wrap error/If Action Subsystem ==
  In1 : Inport
  Action Port : ActionPort  ActionPortLabel=else
  Out1 : Outport
  wires:
  In1/1 -> Out1/1

== system stacked_singleEMRAX_angleChange/Wrap error/Subtract 2pi1 ==
  In1 : Inport
  Action Port : ActionPort  ActionPortLabel=if(u1 > .5)
  Add5 : Sum  Inputs=+-
  Constant2 : Constant
  Out1 : Outport
  wires:
  In1/1 -> Add5/1
  Add5/1 -> Out1/1
  Constant2/1 -> Add5/2

== system stacked_singleEMRAX_angleChange/Wrap error1/Add 2pi ==
  In1 : Inport
  Action Port : ActionPort  ActionPortLabel=elseif(u1<-.5)
  Add5 : Sum
  Constant2 : Constant
  Out1 : Outport
  wires:
  In1/1 -> Add5/1
  Add5/1 -> Out1/1
  Constant2/1 -> Add5/2

== system stacked_singleEMRAX_angleChange/Wrap error1/If Action Subsystem ==
  In1 : Inport
  Action Port : ActionPort  ActionPortLabel=else
  Out1 : Outport
  wires:
  In1/1 -> Out1/1

== system stacked_singleEMRAX_angleChange/Wrap error1/Subtract 2pi1 ==
  In1 : Inport
  Action Port : ActionPort  ActionPortLabel=if(u1 > .5)
  Add5 : Sum  Inputs=+-
  Constant2 : Constant
  Out1 : Outport
  wires:
  In1/1 -> Add5/1
  Add5/1 -> Out1/1
  Constant2/1 -> Add5/2

== system stacked_singleEMRAX_angleChange/Wrap error2/Add 2pi ==
  In1 : Inport
  Action Port : ActionPort  ActionPortLabel=elseif(u1<-.5)
  Add5 : Sum
  Constant2 : Constant
  Out1 : Outport
  wires:
  In1/1 -> Add5/1
  Add5/1 -> Out1/1
  Constant2/1 -> Add5/2

== system stacked_singleEMRAX_angleChange/Wrap error2/If Action Subsystem ==
  In1 : Inport
  Action Port : ActionPort  ActionPortLabel=else
  Out1 : Outport
  wires:
  In1/1 -> Out1/1

== system stacked_singleEMRAX_angleChange/Wrap error2/Subtract 2pi1 ==
  In1 : Inport
  Action Port : ActionPort  ActionPortLabel=if(u1 > .5)
  Add5 : Sum  Inputs=+-
  Constant2 : Constant
  Out1 : Outport
  wires:
  In1/1 -> Add5/1
  Add5/1 -> Out1/1
  Constant2/1 -> Add5/2

== matlab function stacked_singleEMRAX_angleChange/Motor and Propeller/BEMT/MATLAB Function ==
  data: rotorParams input; omega input; Ct output; t input; Cp output; VR_12 input
function [Ct,Cp] = BladeLoop(rotorParams,omega,t,VR_12)
%This function calculates the parameters of individual blade elements 
%neglecting tip loss
%{
Parameters specific to rotor:
rotorParams = [R sigma cla cd c rho mu]
number of elements, n: 20
root cutout: 12%
%}
tol = 1e-3;

R           =   rotorParams(1);                                             % rotor radius [m]
sigma       =   rotorParams(2);                                             % solidity
cla         =   rotorParams(3);                                             % local lift slope [/rad]
cd          =   rotorParams(4);                                             % local drag coefficient
c           =   rotorParams(5);                                             % chord [m]
rho         =   rotorParams(6);                                             % air density [kg/m^3]
mu          =   rotorParams(7);                                             % dynamic viscosity [N-s/m^2]
n           =   20;
R_cutout    =   0.12*R;                                                     % root cutout [m]
R_steps     =   linspace(R_cutout,R*0.9,n)/R;                                 % radial steps [m]
dr          =   (R_steps(2) - R_steps(1))/R;                                    % elemental radius [m]
alpha_table =   VR_12(:,1);
cl_table    =   VR_12(:,2);                                                 % lift values of VR-12 CFD
cd_table    =   VR_12(:,3);                                                 % drag values of VR-12 CFD

    cnt = 1; lambda = 0; alpha = t; %lambda = zeros(n,1); alpha = t*zeros(n,1);                     %first guess is collective position
    ct = zeros(n,1); cpi = zeros(n,1); cpo = zeros(n,1); cp = zeros(n,1);
    for r = R_steps
                
        %Uncomment if wanting to use a VR-12 lookup table 
        [cl0,cd0]       = VR12_lookup_rev3(0,alpha_table,cl_table,cd_table);
        
        %iterate on alpha using VR-12 lookup table
        [cl,cd]         = VR12_lookup_rev3(alpha,alpha_table,cl_table,cd_table);
        
        cla            = 2*(sqrt(2)*sqrt(complex(cl^3*r*sigma - 3*cl^2*r*sigma*cl0 ...
            + 3*cl*r*sigma*cl0^2 - r*sigma*cl0^3)) - 4*cl*r*t + 4*r*t*cl0)/...
            (cl*sigma - 8*r*t^2 - sigma*cl0);
        cla            = real(cla);  %take real part  
        
        lambda    = sigma*cla/16*(sqrt(1 + 32*t*r/sigma/cla) - 1);
        lambda    = real(lambda);
        
        alpha_new       = t - lambda/r;
        while abs(alpha_new-alpha) > tol
            alpha  = alpha_new;
            [cl,cd]    = VR12_lookup_rev3(alpha,alpha_table,cl_table,cd_table);
            
            cla            = 2*(sqrt(2)*sqrt(cl^3*r*sigma - 3*cl^2*r*sigma*cl0 ...
                + 3*cl*r*sigma*cl0^2 - r*sigma*cl0^3) - 4*cl*r*t + 4*r*t*cl0)/...
                (cl*sigma - 8*r*t^2 - sigma*cl0);
            cla            = real(cla);  %take real part
            
            lambda    = sigma*cla/16*(sqrt(1 + 32.*t.*r./sigma./cla) - 1);
            lambda    = real(lambda);

            alpha_new   = t - lambda/r;
        end
        
        if isnan(lambda) 
            lambda = 0;
        end

        %Blade Element Parameters
        ct(cnt)         = 0.5*sigma*cl*r^2*dr; % ct(lambda)
        cpi(cnt)        = ct(cnt)*lambda;
        cpo(cnt)        = 0.5*sigma*r^3*cd*dr;
        cp(cnt)         = cpi(cnt) + cpo(cnt);
        
        cnt = cnt + 1;
    end
    Ct = sum(ct,'omitnan');
    Cp = sum(cp,'omitnan');
end

function [cl,cd] = VR12_lookup_rev3(alpha,alpha_table,cl_table,cd_table)
%{
this function looks up the VR12 airfoil data from 
UT CFD Simulations
Inputs: alpha (Angle of Attack) [rad]
Outputs: cl (local lift coefficient) [-], cd (local drag coefficient) [-]
%}

alpha = alpha*180/pi; % convert to degrees
 
coder.extrinsic('find'); % add find function to simulink function
coder.extrinsic('interp1'); % add interp1 function to simulink function
coder.extrinsic('isempty'); % add isempty function to simulink function

%Find cl and cd
% idx = ones(size(alpha_table,1),1);
% idx = idx.*ismember(alpha_table,alpha); idx = ones(size(alpha_table,1));
check = true(1);
check = isempty(find(alpha_table == alpha));

if check == 0 %there IS an exact AoA in the lookup table
    idx = 0;
    idx = find(alpha_table == alpha);
    cl = cl_table(idx);
    cd = cd_table(idx);
    
else %find the closest AoA in lookup table
    cl = interp1(alpha_table,cl_table,alpha,'linear');
    cd = interp1(alpha_table,cd_table,alpha,'linear');
end

end
